simulink model "Task3"  (R2016a)
settings: Solver=VariableStepAuto  StartTime=0.0  StopTime=10.0  RelTol=1e-3
settings Model: Creator=Thomas  LastModifiedBy=Thomas

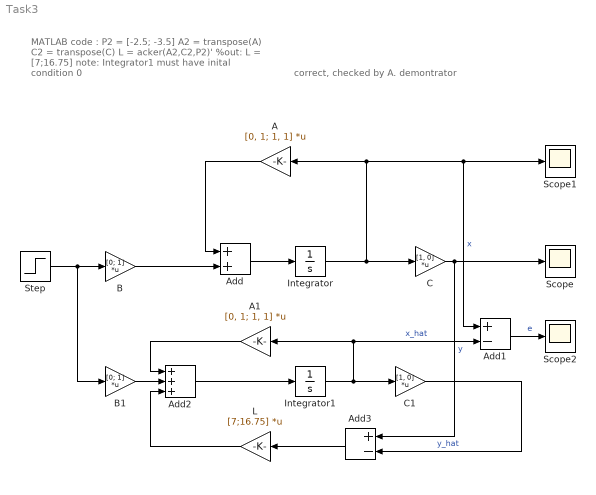
== system Task3 ==
  note: correct, checked by A. demontrator
  note: MATLAB code :
      | P2 = [-2.5; -3.5]
      | A2 = transpose(A)
      | C2 = transpose(C)
      | L = acker(A2,C2,P2)'
      | %out: L = [7;16.75]
      |
      | note: Integrator1 must have inital condition 0
  A : Gain  Gain=[0, 1; 1, 1]  Multiplication=Matrix(K*u)
  A1 : Gain  Gain=[0, 1; 1, 1]  Multiplication=Matrix(K*u)
  Add : Sum
  Add1 : Sum  Inputs=+-
  Add2 : Sum  Inputs=+++
  Add3 : Sum  Inputs=+-
  B : Gain  Gain=[0; 1]  Multiplication=Matrix(K*u)
  B1 : Gain  Gain=[0; 1]  Multiplication=Matrix(K*u)
  C : Gain  Gain=[1, 0]  Multiplication=Matrix(K*u)
  C1 : Gain  Gain=[1, 0]  Multiplication=Matrix(K*u)
  Integrator : Integrator  InitialCondition=[1;1]
  Integrator1 : Integrator
  L : Gain  Gain=[7;16.75]  Multiplication=Matrix(K*u)
  Scope : Scope
  Scope1 : Scope
  Scope2 : Scope
  Step : Step  SampleTime=0
  wires:
  Add/1 -> Integrator/1
  A/1 -> Add/1
  B/1 -> Add/2
  Integrator/1 -> A/1, Add1/1, Scope1/1, C/1  "x"
  C/1 -> Add3/1, Scope/1  "y"
  Step/1 -> B1/1, B/1
  B1/1 -> Add2/2
  A1/1 -> Add2/1
  L/1 -> Add2/3
  Add2/1 -> Integrator1/1
  Integrator1/1 -> A1/1, Add1/2, C1/1  "x_hat"
  Add3/1 -> L/1
  C1/1 -> Add3/2  "y_hat"
  Add1/1 -> Scope2/1  "e"
